simulink model "sampleModel1695_3_sub"  (R2023a)
settings: Solver=VariableStepAuto  StartTime=0.0  StopTime=10.0  RelTol=1e-3
libraries: hdlsllib x3, simulink x3
settings Model: Creator=user1  LastModifiedBy=user1

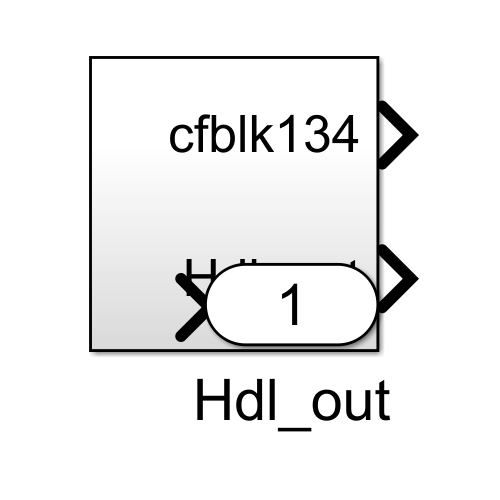
[thumbnail: Simulink's stored preview of the top-level diagram]
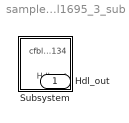
== system sampleModel1695_3_sub ==
  Subsystem : Subsystem
  Hdl_out : Outport  OutDataTypeStr=uint8

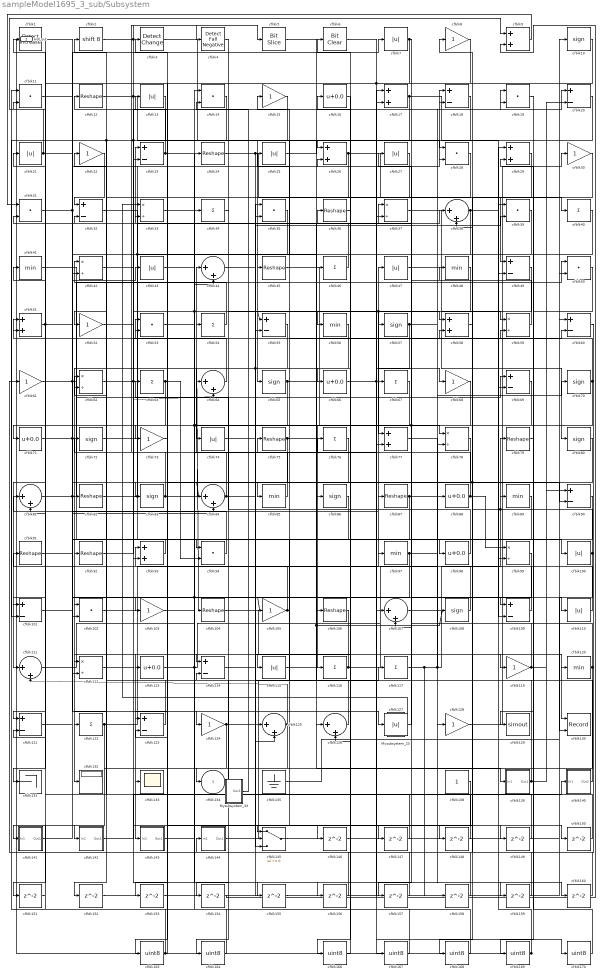
== system sampleModel1695_3_sub/Subsystem ==
  Mysubsystem_23 : Subsystem  TreatAsAtomicUnit=on  RTWFcnName=Mysubsystem_23
      settings: RTWFcnNameOpts=User specified  RTWFileNameOpts=Use function name
  Mysubsystem_33 : Subsystem  TreatAsAtomicUnit=on  RTWFcnName=Mysubsystem_33
      settings: RTWFcnNameOpts=User specified  RTWFileNameOpts=Use function name
  cfblk1 : simulink/Logic and Bit Operations/Detect Increase  vinit=0.0  OutDataTypeStr=uint8
      settings: LibrarySourceBlock=|
      | hdlsllib/Logic and Bit
      | Operations/Detect
      | Increase
  cfblk{10,57,65,70,72,80,83,86,108} (9 alike) : Signum
  cfblk{7,13,21,25,27,43,47,74,100,110,115,127} (12 alike) : Abs  OutDataTypeStr=uint8  SaturateOnIntegerOverflow=off
  cfblk{18,20,23,32,49,55,60,69,90,101,109,114,121,123} (14 alike) : Sum  Inputs=+-  OutDataTypeStr=uint8
  cfblk{11,14,19,28,31,35,39,50,53,94,102} (11 alike) : DotProduct  OutDataTypeStr=uint8
  cfblk{8,15,22,30,52,61,68,73,103,105,119,124,128} (13 alike) : Gain  OutDataTypeStr=uint8
  cfblk{12,24,36,45,75,79,82,87,91..92,104,106} (12 alike) : Reshape
  cfblk{38,44,64,81,84,107,111,125..126} (9 alike) : Sum  Inputs=|++  OutDataTypeStr=uint8
  cfblk{33,37,42,59,62,78,99,112} (8 alike) : Product  Inputs=*/  OutDataTypeStr=uint8  RndMeth=Zero  SaturateOnIntegerOverflow=on
  cfblk{16,66,71,88,98,113} (6 alike) : Bias  Bias=0.0  SaturateOnIntegerOverflow=off
  cfblk{34,40,46,54,63,67,76,116..117,122} (10 alike) : Sum  Inputs=+  OutDataTypeStr=uint8
  cfblk{41,48,56,85,89,97,120} (7 alike) : MinMax  OutDataTypeStr=uint8
  cfblk129 : ToWorkspace  VariableName=simout  SaveFormat=Timeseries  SampleTime=-1
  cfblk130 : Record  FileSettingsInternal="{\"entries\":[{\"content\":{\"excelSettings\":{\"content\":{},\"type\":\"Streamout.ExcelSettings\"}},\"type\":\"Streamout.FileSettingStorage\",\"uuid\":\"\"}],\"packageUris\":[\"http:\\/\\/schema.mathworks.com\\/mf0\\/streamout_blocks\\/R2020a\"],\"version\":\"1.0\"}"  Layout=[1 1]  SignalsInternal="{\"entries\":[{\"content\":{\"signals\":[{\"content\":{\"blockPath\":[],\"dimensions\":[1],\"domain\":\"\",\"lineColor\":\"#a2142f\",\"plots\":[1],\"port\":1,\"signalID\":35563,\"signalName\":\"cfblk104\"},\"type\":\"RecordBlkView.Signal\",\"uuid\":\"\"},{\"content\":{\"blockPath\":[],\"dimensions\":[1],\"domain\":\"\",\"lineColor\":\"#139fff\",\"plots\":[1],\"port\":2,\"signalID\":35566,\"signalName\":\"cfblk100\"},\"type\":\"RecordBlkView.Signal\",\"uuid\":\"\"}]},\"type\":\"RecordBlkView.InputSignals\",\"uuid\":\"\"}],\"packageUris\":[\"http:\\/\\/schema.mathworks.com\\/mf0\\/streamout_blocks\\/R2020a\"],\"version\":\"1.0\"}"  VisualizationBindings="{\"xyplotplugin\":{\"info\":[{\"series\":[{\"bindingParametersList\":[{\"parameter\":\"X-Axis\",\"signalID\":35563,\"signalName\":\"cfblk104\"},{\"parameter\":\"Y-Axis\",\"signalID\":35566,\"signalName\":\"cfblk100\"}],\"seriesID\":28457}],\"subplotID\":1}]}}"  CompatibilityTag=XY  st=-1
  cfblk131 : Terminator
  cfblk132 : Display
  cfblk133 : Scope
  cfblk135 : Ground
  cfblk138 : Constant  OutDataTypeStr=uint8  SampleTime=-1
  cfblk139 : Subsystem
      settings: LibrarySourceBlock=|
      | hdlsllib/Ports &
      | Subsystems/Subsystem
  cfblk140 : Subsystem
      settings: LibrarySourceBlock=|
      | hdlsllib/Ports &
      | Subsystems/Subsystem
  cfblk141 : Subsystem
      settings: LibrarySourceBlock=|
      | hdlsllib/Ports &
      | Subsystems/Subsystem
  cfblk142 : Subsystem
      settings: LibrarySourceBlock=|
      | hdlsllib/Ports &
      | Subsystems/Subsystem
  cfblk143 : Subsystem
      settings: LibrarySourceBlock=|
      | hdlsllib/Ports &
      | Subsystems/Subsystem
  cfblk144 : Subsystem
      settings: LibrarySourceBlock=|
      | hdlsllib/Ports &
      | Subsystems/Subsystem
  cfblk145 : Switch  OutDataTypeStr=uint8  SaturateOnIntegerOverflow=off  InputSameDT=off
  cfblk{146..160} (15 alike) : Delay  SampleTime=1
  cfblk{163..164,166..170} (7 alike) : DataTypeConversion  OutDataTypeStr=uint8  SaturateOnIntegerOverflow=off  RndMeth=Floor
  cfblk{9,17,26,29,51,58,77,93} (8 alike) : Sum  OutDataTypeStr=uint8
  cfblk2 : ArithShift  BitShiftNumber=8
  cfblk3 : simulink/Logic and Bit Operations/Detect Change  vinit=0  OutDataTypeStr=uint8
      settings: LibrarySourceBlock=|
      | hdlsllib/Logic and Bit
      | Operations/Detect
      | Change
  cfblk4 : hdlsllib/Logic and Bit Operations/Detect Fall Negative  vinit=0  OutDataTypeStr=uint8
  cfblk5 : hdlsllib/Logic and Bit Operations/Bit Slice  lidx=7  ridx=0
  cfblk6 : simulink/Logic and Bit Operations/Bit Clear  iBit=0
      settings: LibrarySourceBlock=|
      | hdlsllib/Logic and Bit
      | Operations/Bit Clear
  cfblk134 : Outport  OutDataTypeStr=uint8  VectorParamsAs1DForOutWhenUnconnected=off
  Hdl_out : Outport  Port=2  OutDataTypeStr=uint8
  wires:
  cfblk87/1 -> cfblk149/1, cfblk132/1
  cfblk119/1 -> cfblk20/2, cfblk93/1
  cfblk126/1 -> cfblk3/1
  cfblk83/1 -> cfblk17/2, cfblk5/1
  cfblk50/1 -> cfblk115/1
  cfblk85/1 -> cfblk44/1
  cfblk125/1 -> cfblk111/2, cfblk141/1(In1)
  cfblk106/1 -> cfblk143/1(In1)
  cfblk102/1 -> cfblk47/1
  cfblk3/1 -> cfblk26/1
  cfblk107/1 -> cfblk110/1
  cfblk41/1 -> cfblk98/1
  cfblk81/1 -> cfblk99/2, cfblk50/1
  cfblk54/1 -> cfblk42/1
  cfblk46/1 -> cfblk23/1
  cfblk124/1 -> cfblk117/1, cfblk134/1
  cfblk139/1(Out1) -> cfblk90/1, cfblk75/1
  cfblk88/1 -> cfblk99/1, cfblk2/1
  cfblk53/1 -> cfblk34/1
  cfblk48/1 -> cfblk126/2, cfblk77/1
  cfblk145/1 -> cfblk50/2
  cfblk39/1 -> cfblk42/2
  cfblk56/1 -> cfblk102/1
  cfblk128/1 -> cfblk30/1
  cfblk138/1 -> cfblk61/1
  cfblk127/1 -> cfblk57/1
  cfblk140/1(Out1) -> cfblk62/1
  cfblk51/1 -> cfblk83/1, cfblk111/1
  cfblk89/1 -> cfblk102/2
  cfblk8/1 -> cfblk93/2
  cfblk57/1 -> cfblk19/2, cfblk67/1
  cfblk62/1 -> cfblk54/1, cfblk18/1
  cfblk68/1 -> cfblk116/1
  cfblk117/1 -> cfblk158/1, cfblk70/1, cfblk79/1
  cfblk45/1 -> cfblk78/1
  cfblk55/1 -> cfblk145/2, cfblk104/1
  cfblk16/1 -> cfblk66/1
  cfblk58/1 -> cfblk8/1
  cfblk26/1 -> cfblk73/1, cfblk40/1
  cfblk60/1 -> cfblk144/1(In1)
  cfblk72/1 -> cfblk36/1
  cfblk30/1 -> cfblk49/1
  cfblk123/1 -> cfblk22/1
  cfblk21/1 -> cfblk124/1, cfblk9/1
  cfblk70/1 -> cfblk25/1, cfblk81/2, cfblk74/1
  cfblk37/1 -> cfblk59/1
  cfblk76/1 -> cfblk86/1
  cfblk144/1(Out1) -> cfblk46/1
  cfblk86/1 -> cfblk145/1
  cfblk28/1 -> cfblk56/1
  cfblk32/1 -> cfblk126/1, cfblk106/1
  cfblk7/1 -> cfblk107/2, cfblk37/2, cfblk133/1
  cfblk23/1 -> cfblk156/1, cfblk12/1
  cfblk103/1 -> cfblk76/1
  cfblk122/1 -> cfblk151/1, cfblk97/1
  cfblk110/1 -> cfblk53/1
  cfblk116/1 -> cfblk112/1, cfblk78/2
  cfblk67/1 -> cfblk123/1
  cfblk64/1 -> cfblk51/1
  cfblk66/1 -> cfblk170/1, cfblk68/1
  cfblk101/1 -> cfblk43/1
  cfblk104/1 -> cfblk130/1
  cfblk63/1 -> cfblk94/2, cfblk82/1
  cfblk15/1 -> cfblk23/2, cfblk131/1
  cfblk120/1 -> cfblk31/2, cfblk142/1(In1)
  cfblk52/1 -> cfblk26/2
  cfblk10/1 -> cfblk71/1
  cfblk97/1 -> cfblk112/2, cfblk19/1
  cfblk12/1 -> cfblk155/1, cfblk65/1
  cfblk82/1 -> cfblk145/3, cfblk24/1
  cfblk142/1(Out1) -> cfblk140/1(In1)
  cfblk93/1 -> cfblk92/1
  cfblk25/1 -> cfblk28/1
  cfblk9/1 -> cfblk31/1
  cfblk80/1 -> cfblk148/1, cfblk84/1
  cfblk69/1 -> cfblk147/1, cfblk94/1
  cfblk22/1 -> cfblk32/1
  cfblk71/1 -> cfblk85/1, cfblk69/1
  cfblk109/1 -> cfblk91/1
  cfblk27/1 -> cfblk52/1
  cfblk47/1 -> cfblk80/1
  cfblk1/1 -> cfblk84/2, cfblk121/1
  cfblk40/1 -> cfblk122/1
  cfblk98/1 -> cfblk63/1
  cfblk65/1 -> cfblk139/1(In1), cfblk101/1
  cfblk17/1 -> cfblk103/1, cfblk69/2
  cfblk43/1 -> cfblk18/2
  cfblk94/1 -> cfblk21/1
  cfblk105/1 -> cfblk81/1, cfblk15/1
  cfblk92/1 -> cfblk20/1
  cfblk14/1 -> cfblk163/1
  cfblk59/1 -> cfblk27/1
  cfblk18/1 -> cfblk45/1
  cfblk75/1 -> cfblk153/1, cfblk59/2
  cfblk100/1 -> cfblk130/2, cfblk48/1, cfblk89/1
  cfblk73/1 -> cfblk13/1
  cfblk5/1 -> cfblk119/1
  cfblk111/1 -> cfblk44/2
  cfblk113/1 -> cfblk58/2, cfblk88/1
  cfblk11/1 -> cfblk109/1
  cfblk115/1 -> cfblk37/1, cfblk108/1
  cfblk2/1 -> cfblk64/2, cfblk4/1
  cfblk44/1 -> cfblk39/2
  cfblk24/1 -> cfblk109/2, cfblk125/1
  cfblk74/1 -> cfblk120/1
  cfblk38/1 -> cfblk55/2, cfblk49/2
  cfblk143/1(Out1) -> cfblk38/1
  cfblk135/1 -> cfblk10/1
  cfblk79/1 -> cfblk129/1
  cfblk121/1 -> cfblk127/1
  cfblk13/1 -> cfblk152/1, cfblk101/2
  cfblk61/1 -> cfblk100/1, cfblk128/1
  cfblk49/1 -> cfblk114/1
  cfblk31/1 -> cfblk90/2, cfblk28/2
  cfblk33/1 -> cfblk55/1, cfblk77/2, cfblk159/1, cfblk105/1
  cfblk108/1 -> cfblk62/2
  cfblk91/1 -> cfblk87/1
  cfblk34/1 -> cfblk64/1
  cfblk42/1 -> cfblk58/1
  cfblk36/1 -> cfblk16/1
  cfblk141/1(Out1) -> cfblk7/1
  cfblk84/1 -> cfblk60/2, cfblk72/1
  cfblk114/1 -> cfblk35/2
  cfblk35/1 -> cfblk113/1
  cfblk20/1 -> cfblk146/1
  cfblk146/1 -> cfblk39/1
  cfblk147/1 -> cfblk1/1
  cfblk148/1 -> cfblk51/2
  cfblk149/1 -> cfblk114/2
  cfblk112/1 -> cfblk150/1
  cfblk150/1 -> cfblk32/2
  cfblk151/1 -> cfblk121/2
  cfblk152/1 -> cfblk107/1
  cfblk153/1 -> cfblk125/2
  cfblk90/1 -> cfblk154/1
  cfblk154/1 -> cfblk9/2
  cfblk155/1 -> cfblk60/1
  cfblk156/1 -> cfblk123/2
  cfblk99/1 -> cfblk157/1
  cfblk157/1 -> cfblk17/1
  cfblk158/1 -> cfblk53/2
  cfblk159/1 -> cfblk38/2
  cfblk77/1 -> cfblk160/1
  cfblk160/1 -> cfblk35/1
  cfblk163/1 -> cfblk41/1, cfblk33/2
  cfblk4/1 -> cfblk164/1
  cfblk164/1 -> cfblk14/1
  cfblk78/1 -> cfblk166/1
  cfblk166/1 -> cfblk6/1
  cfblk6/1 -> cfblk167/1
  cfblk167/1 -> cfblk11/2
  cfblk29/1 -> cfblk168/1
  cfblk168/1 -> cfblk11/1
  cfblk19/1 -> cfblk169/1
  cfblk169/1 -> Hdl_out/1, cfblk29/1
  cfblk170/1 -> cfblk29/2
  Mysubsystem_23/1(Out1) -> cfblk33/1
  Mysubsystem_33/1(Out1) -> cfblk14/2

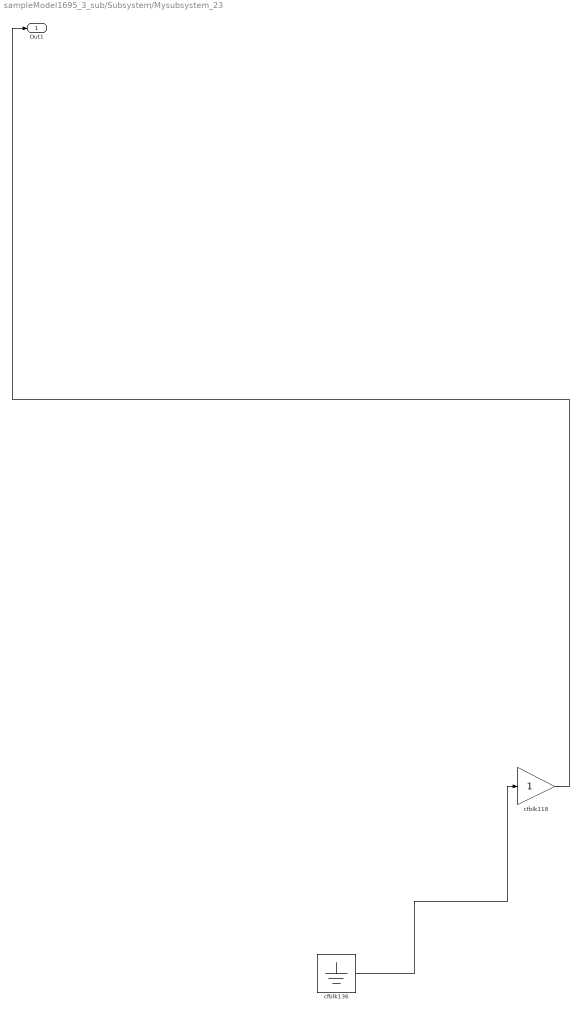
== system sampleModel1695_3_sub/Subsystem/Mysubsystem_23 ==
  cfblk118 : Gain
  cfblk136 : Ground
  Out1 : Outport
  wires:
  cfblk118/1 -> Out1/1
  cfblk136/1 -> cfblk118/1

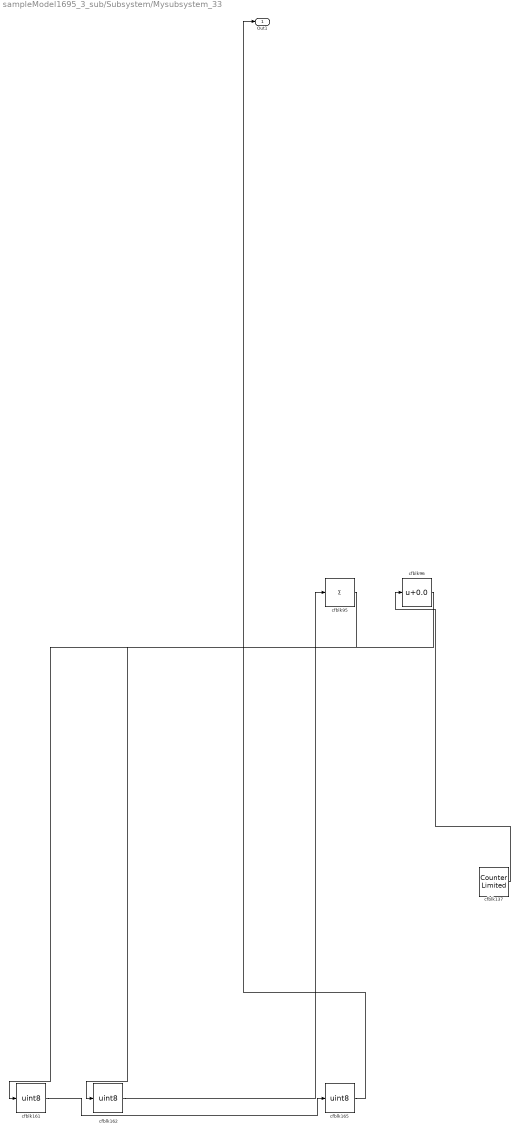
== system sampleModel1695_3_sub/Subsystem/Mysubsystem_33 ==
  cfblk137 : hdlsllib/Sources/Counter Limited  uplimit=7  tsamp=-1
  cfblk161 : DataTypeConversion  OutDataTypeStr=uint8  SaturateOnIntegerOverflow=off  RndMeth=Floor
  cfblk162 : DataTypeConversion  OutDataTypeStr=uint8  SaturateOnIntegerOverflow=off  RndMeth=Floor
  cfblk165 : DataTypeConversion  OutDataTypeStr=uint8  SaturateOnIntegerOverflow=off  RndMeth=Floor
  cfblk95 : Sum  Inputs=+
  cfblk96 : Bias  Bias=0.0  SaturateOnIntegerOverflow=off
  Out1 : Outport
  wires:
  cfblk165/1 -> Out1/1
  cfblk162/1 -> cfblk95/1
  cfblk137/1 -> cfblk96/1
  cfblk161/1 -> cfblk165/1
  cfblk96/1 -> cfblk162/1
  cfblk95/1 -> cfblk161/1

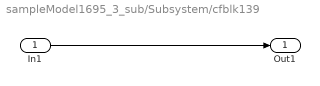
== system sampleModel1695_3_sub/Subsystem/cfblk139 ==
  In1 : Inport
  Out1 : Outport
  wires:
  In1/1 -> Out1/1

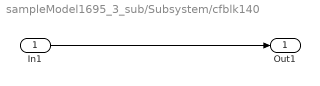
== system sampleModel1695_3_sub/Subsystem/cfblk140 ==
  In1 : Inport
  Out1 : Outport
  wires:
  In1/1 -> Out1/1

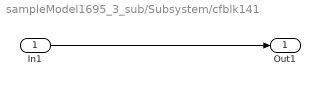
== system sampleModel1695_3_sub/Subsystem/cfblk141 ==
  In1 : Inport
  Out1 : Outport
  wires:
  In1/1 -> Out1/1

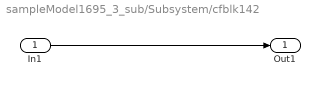
== system sampleModel1695_3_sub/Subsystem/cfblk142 ==
  In1 : Inport
  Out1 : Outport
  wires:
  In1/1 -> Out1/1

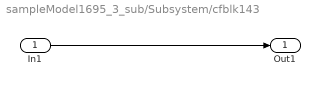
== system sampleModel1695_3_sub/Subsystem/cfblk143 ==
  In1 : Inport
  Out1 : Outport
  wires:
  In1/1 -> Out1/1

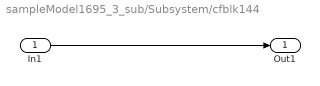
== system sampleModel1695_3_sub/Subsystem/cfblk144 ==
  In1 : Inport
  Out1 : Outport
  wires:
  In1/1 -> Out1/1
